simulink model "scenarioCloseLoop_supervisoryACC_start"  (R2019b)
settings: Solver=VariableStepAuto  StartTime=0.0  StopTime=30  FixedStep=0.01  RelTol=1e-3
PreLoadFcn:
  | Ts1 = -1;
  | Ts2 = -1;
InitFcn:
  | initACCParams_pid;
model workspace (MAT data in the model file):
  firstWarning = 1
  originalScenarioChecksum = '3C3E23DDE530CB8BEC76DD6DBB66960A'
undefined symbols (not defined in the file): APP_gain, BPP_gain, default_spacing, DiscIntNeverNeededParam, m, sigbuilder_block, steer_gain, time_gap
libraries: drivingscenarioandsensors x2, simulink x1, autolibshared x1, vehdynlibviscommon x1
settings Model: EnablePacing=on  Creator=sseshadr  LastModifiedBy=cdsouza
settings SolverCC: AutoInsertRateTranBlk=on
settings OptimizationCC: DefaultParameterBehavior=Inlined  EnhancedBackFolding=on  PassReuseOutputArgsThreshold=0  OptimizeBlockOrder=speed  DifferentSizesBufferReuse=on  OptimizationCustomize=off
settings DebuggingCC: ParameterTunabilityLossMsg=error
settings SFSimCC: MATLABDynamicMemAlloc=off
settings RTWCC: Description=Generic Real-Time Target  GenerateReport=on  LaunchReport=on
settings CodeAppCC: ForceParamTrailComments=on  OperatorAnnotations=on  StateflowObjectComments=on

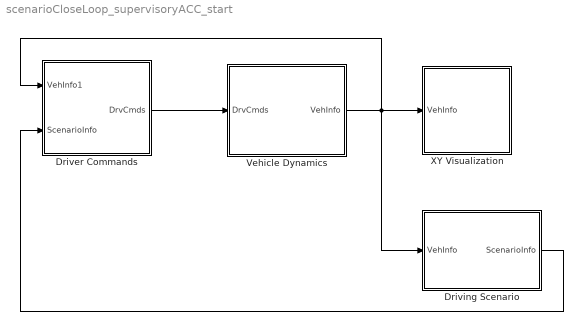
== system scenarioCloseLoop_supervisoryACC_start ==
  Driver Commands : Subsystem
  Driving Scenario : Subsystem
  Vehicle Dynamics : Subsystem
  XY Visualization : Subsystem
  wires:
  Driving Scenario/1(ScenarioInfo) -> Driver Commands/2(ScenarioInfo)
  Driver Commands/1(DrvCmds) -> Vehicle Dynamics/1(DrvCmds)
  Vehicle Dynamics/1(VehInfo) -> Driving Scenario/1(VehInfo), XY Visualization/1(VehInfo), Driver Commands/1(VehInfo1)

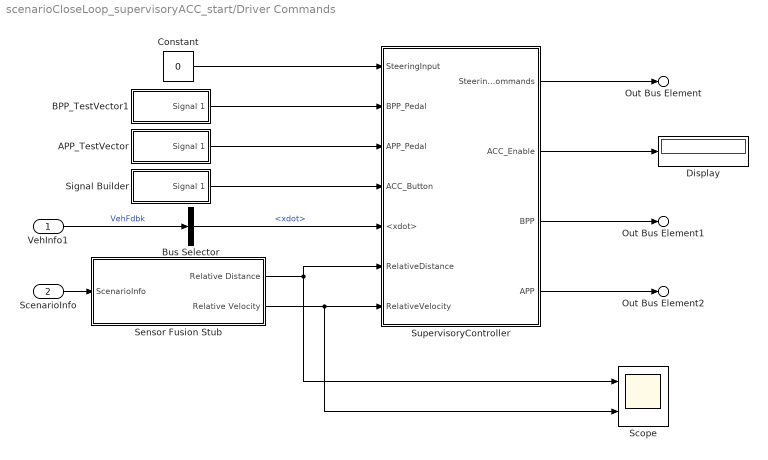
== system scenarioCloseLoop_supervisoryACC_start/Driver Commands ==
  VehInfo1 : Inport
  ScenarioInfo : Inport  Port=2
  APP_TestVector : Subsystem  Tag=STV Subsys  LoadFcn=sigbuilder_block('load');  StartFcn=sigbuilder_block('start');  StopFcn=sigbuilder_block('stop');  ClipboardFcn=sigbuilder_block('clipboard');  mask(Sigbuilder block){tuvar=[0:10]}
      mask help: Simulink:masks:SigbuilderBlock_MD
      mask init:
      | if ~strcmp(get_param(bdroot(gcbh),'SimulationStatus'),'stopped') tuvar = sigbuilder_block('maskInit'); end
      settings: CopyFcn=sigbuilder_block('copy');  DeleteFcn=sigbuilder_block('delete');  ModelCloseFcn=sigbuilder_block('modelClose');  PreSaveFcn=sigbuilder_block('preSave');  PauseFcn=sigbuilder_block('pause');  ContinueFcn=sigbuilder_block('continue');  NameChangeFcn=sigbuilder_block('namechange');  OpenFcn=sigbuilder_block('open',[609 515.25 550.5 237.75 ]);  CloseFcn=sigbuilder_block('close');
      mask Display: plot(0, 0, 100, 100,[2, 2, 32, 32, 2], [68, 8, 8, 68, 68],[32, 2], [38, 38], [32, 19, 2],[53, 60, 44], [32, 17, 17, 2],[16, 16, 31, 31]);txt = getActiveGroup(gcbh);text(2, 100, txt,'verticalAlignment', 'top');
  BPP_TestVector1 : Subsystem  Tag=STV Subsys  LoadFcn=sigbuilder_block('load');  StartFcn=sigbuilder_block('start');  StopFcn=sigbuilder_block('stop');  ClipboardFcn=sigbuilder_block('clipboard');  mask(Sigbuilder block){tuvar=[0:10]}
      mask help: Simulink:masks:SigbuilderBlock_MD
      mask init:
      | if ~strcmp(get_param(bdroot(gcbh),'SimulationStatus'),'stopped') tuvar = sigbuilder_block('maskInit'); end
      settings: CopyFcn=sigbuilder_block('copy');  DeleteFcn=sigbuilder_block('delete');  ModelCloseFcn=sigbuilder_block('modelClose');  PreSaveFcn=sigbuilder_block('preSave');  PauseFcn=sigbuilder_block('pause');  ContinueFcn=sigbuilder_block('continue');  NameChangeFcn=sigbuilder_block('namechange');  OpenFcn=sigbuilder_block('open',[325.5 304.5 550.5 278.25 ]);  CloseFcn=sigbuilder_block('close');
      mask Display: plot(0, 0, 100, 100,[2, 2, 32, 32, 2], [68, 8, 8, 68, 68],[32, 2], [38, 38], [32, 19, 2],[53, 60, 44], [32, 17, 17, 2],[16, 16, 31, 31]);txt = getActiveGroup(gcbh);text(2, 100, txt,'verticalAlignment', 'top');
  Bus Selector : BusSelector  OutputSignals=BdyFrm.Cg.Vel.xdot
  Constant : Constant  Value=0  SampleTime=0.01
  Display : Display
  Scope : Scope  NumInputPorts=2
  Sensor Fusion Stub : Subsystem
  Signal Builder : Subsystem  Tag=STV Subsys  LoadFcn=sigbuilder_block('load');  StartFcn=sigbuilder_block('start');  StopFcn=sigbuilder_block('stop');  ClipboardFcn=sigbuilder_block('clipboard');  mask(Sigbuilder block){tuvar=[0:10]}
      mask help: Simulink:masks:SigbuilderBlock_MD
      mask init:
      | if ~strcmp(get_param(bdroot(gcbh),'SimulationStatus'),'stopped') tuvar = sigbuilder_block('maskInit'); end
      settings: CopyFcn=sigbuilder_block('copy');  DeleteFcn=sigbuilder_block('delete');  ModelCloseFcn=sigbuilder_block('modelClose');  PreSaveFcn=sigbuilder_block('preSave');  PauseFcn=sigbuilder_block('pause');  ContinueFcn=sigbuilder_block('continue');  NameChangeFcn=sigbuilder_block('namechange');  OpenFcn=sigbuilder_block('open',[401.25 280.5 550.5 278.25 ]);  CloseFcn=sigbuilder_block('close');
      mask Display: plot(0, 0, 100, 100,[2, 2, 32, 32, 2], [68, 8, 8, 68, 68],[32, 2], [38, 38], [32, 19, 2],[53, 60, 44], [32, 17, 17, 2],[16, 16, 31, 31]);txt = getActiveGroup(gcbh);text(2, 100, txt,'verticalAlignment', 'top');
  SupervisoryController : Subsystem
  Out Bus Element : Outport  PortName=DrvCmds  Element=SteerCmd
  Out Bus Element1 : Outport  PortName=DrvCmds  Element=BPP Pedal
  Out Bus Element2 : Outport  PortName=DrvCmds  Element=APP Pedal
  wires:
  ScenarioInfo/1 -> Sensor Fusion Stub/1(ScenarioInfo)
  Sensor Fusion Stub/1(Relative Distance) -> SupervisoryController/6(RelativeDistance), Scope/1
  Sensor Fusion Stub/2(Relative Velocity) -> Scope/2, SupervisoryController/7(RelativeVelocity)
  SupervisoryController/1(SteeringCommands) -> Out Bus Element/1
  SupervisoryController/2(ACC_Enable) -> Display/1
  SupervisoryController/3(BPP) -> Out Bus Element1/1
  SupervisoryController/4(APP) -> Out Bus Element2/1
  Bus Selector/1 -> SupervisoryController/5(<xdot>)  "<xdot>"
  VehInfo1/1 -> Bus Selector/1  "VehFdbk"
  Signal Builder/1(Signal 1) -> SupervisoryController/4(ACC_Button)
  Constant/1 -> SupervisoryController/1("SteeringInput ")
  BPP_TestVector1/1(Signal 1) -> SupervisoryController/2(BPP_Pedal)
  APP_TestVector/1(Signal 1) -> SupervisoryController/3(APP_Pedal)

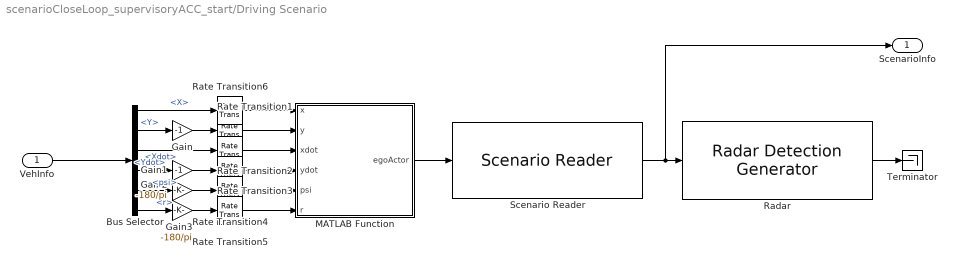
== system scenarioCloseLoop_supervisoryACC_start/Driving Scenario ==
  VehInfo : Inport
  Bus Selector : BusSelector  OutputSignals=InertFrm.Cg.Disp.X,InertFrm.Cg.Disp.Y,InertFrm.Cg.Vel.Xdot,InertFrm.Cg.Vel.Ydot,InertFrm.Cg.Ang.psi,BdyFrm.Cg.AngVel.r
  Gain : Gain  Gain=-1
  Gain1 : Gain  Gain=-1
  Gain2 : Gain  Gain=-180/pi
  Gain3 : Gain  Gain=-180/pi
  MATLAB Function : MATLAB Function  TreatAsAtomicUnit=on
  Radar : drivingscenarioandsensors/Radar Detection Generator  SensorIndex=1  UpdateInterval=0.1  SensorLocation=[3.5 0]  Height=0.2  Yaw=0  Pitch=0  Roll=0  BusNameSource=Auto  BusName=BusRadarDetectionGenerator  MaxNumDetectionsSource=Property  MaxNumDetections=50  DetectionCoordinates=Ego Cartesian  SimulateUsing=Interpreted execution  AzimuthResolution=4  ElevationResolution=10  RangeResolution=2.5  RangeRateResolution=0.5  AzimuthBiasFraction=0.1  ElevationBiasFraction=0.1  RangeBiasFraction=0.05  RangeRateBiasFraction=0.05  FieldOfView=[100 5]  MaxRange=50  RangeRateLimits=[-100 100]  DetectionProbability=0.9  FalseAlarmRate=1e-06  ReferenceRange=100  ReferenceRCS=0  HasElevation=off  HasRangeRate=on  HasNoise=on  HasFalseAlarms=on  HasOcclusion=on  InitialSeedSource=Repeatable  InitialSeed=0  UsedSeed=0  ActorProfilesSource=MATLAB expression  ActorProfilesParameters=driving.internal.ActorProfilesRadarParameters  ActorProfilesExpression=[struct('ActorID',1,'ClassID',1,'Length',4.7,'Width',1.8,'Height',1.4,'OriginOffset',[-1.35 0 0],'RCSPattern',[10 10;10 10],'RCSAzimuthAngles',[-180 180],'RCSElevationAngles',[-90 90]); struct('ActorID',2,'ClassID',1,'Length',4.7,'Width',1.8,'Height',1.4,'OriginOffset',[-1.35 0 0],'RCSPattern',[10 10;10 10],'RCSAzimuthAngles',[-180 180],'RCSElevationAngles',[-90 90]); struct('ActorID',3,'ClassID',1,'Length',4.7,'Width',1.8,'Height',1.4,'OriginOffset',[-1.35 0 0],'RCSPattern',[10 10;10 10],'RCSAzimuthAngles',[-180 180],'RCSElevationAngles',[-90 90]); struct('ActorID',4,'ClassID',1,'Length',4.7,'Width',1.8,'Height',1.4,'OriginOffset',[-1.35 0 0],'RCSPattern',[10 10;10 10],'RCSAzimuthAngles',[-180 180],'RCSElevationAngles',[-90 90])]
      settings: SourceProductName=Automated Driving Toolbox  SourceProductBaseCode=DR
  Rate Transition{1..6} (6 alike) : RateTransition  OutPortSampleTime=0.1
  Scenario Reader : drivingscenarioandsensors/Scenario Reader  ScenarioSource=From file  ScenarioFileName=Straight.mat  ScenarioVariableName=scenario  OutputCoordinateSystem=Vehicle coordinates  EgoVehicleSource=Input port  EgoVehicleActorID=1  SampleTime=0.1  LaneBoundaryOutput=None  LaneBoundaryDistance=0:0.5:9.5  LaneBoundaryLocation=Center of lane markings  BusNameSource=Auto  BusName=BusActors  BusName2Source=Auto  BusName2=BusLaneBoundaries  SimulateUsing=Interpreted execution
      settings: SourceProductName=Automated Driving Toolbox
  Terminator : Terminator
  ScenarioInfo : Outport
  wires:
  Bus Selector/3 -> Rate Transition2/1  "<Xdot>"
  Bus Selector/6 -> Gain3/1  "<r>"
  Bus Selector/1 -> Rate Transition6/1  "<X>"
  Bus Selector/2 -> Gain/1  "<Y>"
  Bus Selector/5 -> Gain2/1  "<psi>"
  VehInfo/1 -> Bus Selector/1
  Bus Selector/4 -> Gain1/1  "<Ydot>"
  Rate Transition6/1 -> MATLAB Function/1(x)
  Rate Transition1/1 -> MATLAB Function/2(y)
  Rate Transition2/1 -> MATLAB Function/3(xdot)
  Rate Transition3/1 -> MATLAB Function/4(ydot)
  Rate Transition4/1 -> MATLAB Function/5(psi)
  Rate Transition5/1 -> MATLAB Function/6(r)
  Radar/1 -> Terminator/1
  Scenario Reader/1 -> ScenarioInfo/1, Radar/1
  MATLAB Function/1(egoActor) -> Scenario Reader/1
  Gain/1 -> Rate Transition1/1
  Gain1/1 -> Rate Transition3/1
  Gain2/1 -> Rate Transition4/1
  Gain3/1 -> Rate Transition5/1

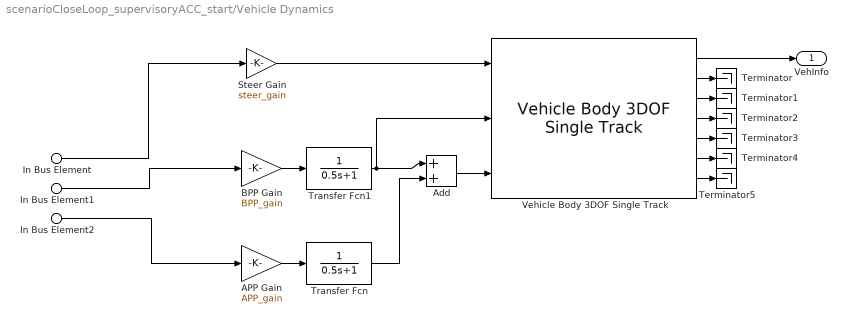
== system scenarioCloseLoop_supervisoryACC_start/Vehicle Dynamics ==
  In Bus Element : Inport  PortName=DrvCmds  Element=SteerCmd
  In Bus Element1 : Inport  PortName=DrvCmds  Element=BPP Pedal
  In Bus Element2 : Inport  PortName=DrvCmds  Element=APP Pedal
  APP Gain : Gain  Gain=APP_gain
  Add : Sum
  BPP Gain : Gain  Gain=BPP_gain
  Steer Gain : Gain  Gain=steer_gain
  Terminator{,1..5} (6 alike) : Terminator
  Transfer Fcn : TransferFcn  Denominator=[0.5 1]
  Transfer Fcn1 : TransferFcn  Denominator=[0.5 1]
  Vehicle Body 3DOF Single Track : autolibshared/Vehicle Body 3DOF Single Track  trackMode=Single (bicycle)  inputMode=External longitudinal forces  frontSteerMode=on  rearSteerMode=off  windMode=off  muMode=off  extFMode=off  extMMode=off  extXo=off  extpsio=off  extxdoto=off  extro=off  extYo=off  extTamb=off  extydoto=off  aMode=2  NF=2  NR=2  m=m  a=1.4  b=1.6  h=0.35  X_o=0  xdot_o=0  CalphaMode=off  sigmaMode=on  d=0  w=[1.4,1.4]  Cy_f=12e3  Cy_r=11e3  sigma_f=.1  sigma_r=.1  alpha_f_brk=[-.1 .1]  Cy_f_data=[-9e3 9e3]  alpha_r_brk=[-.1 .1]  Cy_r_data=[-9e3 9e3]  Y_o=0  ydot_o=0  Izz=4000  psi_o=0  r_o=0  Af=2  Cd=.3  Cl=.1  Cpm=.1  beta_w=[0:0.01:0.3]  Cs=[0:0.03:0.9]  Cym=[0:0.01:0.3]  Pabs=101325  Tair=273  g=9.81  mu=1  xdot_tol=.01  Fznom=5000  Fxtire_sat=7e4  Fytire_sat=7e4  longOff=0  latOff=0  vertOff=0  wrapAng=off
      settings: SourceProductName=Powertrain Blockset  SourceProductBaseCode=PW
  VehInfo : Outport
  wires:
  Vehicle Body 3DOF Single Track/7 -> Terminator5/1
  Transfer Fcn/1 -> Add/2
  Vehicle Body 3DOF Single Track/6 -> Terminator4/1
  BPP Gain/1 -> Transfer Fcn1/1
  In Bus Element1/1 -> BPP Gain/1
  Steer Gain/1 -> Vehicle Body 3DOF Single Track/1
  Vehicle Body 3DOF Single Track/4 -> Terminator2/1
  Vehicle Body 3DOF Single Track/2 -> Terminator/1
  Vehicle Body 3DOF Single Track/5 -> Terminator3/1
  Transfer Fcn1/1 -> Vehicle Body 3DOF Single Track/2, Add/1
  APP Gain/1 -> Transfer Fcn/1
  Vehicle Body 3DOF Single Track/3 -> Terminator1/1
  Add/1 -> Vehicle Body 3DOF Single Track/3
  Vehicle Body 3DOF Single Track/1 -> VehInfo/1
  In Bus Element/1 -> Steer Gain/1
  In Bus Element2/1 -> APP Gain/1

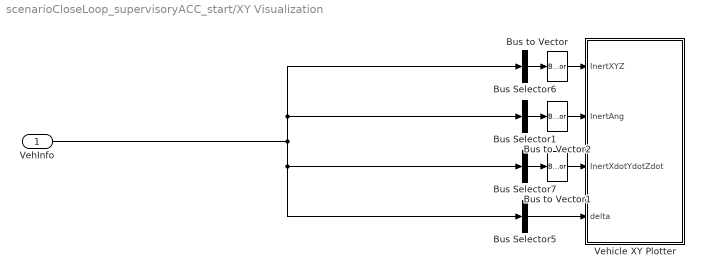
== system scenarioCloseLoop_supervisoryACC_start/XY Visualization ==
  VehInfo : Inport
  Bus Selector1 : BusSelector  OutputSignals=InertFrm.Cg.Ang.phi,InertFrm.Cg.Ang.theta,InertFrm.Cg.Ang.psi  OutputAsBus=on
  Bus Selector5 : BusSelector  OutputSignals=BdyFrm.FrntAxl.Steer.WhlAngFL,BdyFrm.FrntAxl.Steer.WhlAngFR,BdyFrm.RearAxl.Steer.WhlAngRL,BdyFrm.RearAxl.Steer.WhlAngRR  OutputAsBus=on
  Bus Selector6 : BusSelector  OutputSignals=InertFrm.Geom.Disp.X,InertFrm.Geom.Disp.Y,InertFrm.Geom.Disp.Z  OutputAsBus=on
  Bus Selector7 : BusSelector  OutputSignals=InertFrm.Geom.Vel.Xdot,InertFrm.Geom.Vel.Ydot,InertFrm.Geom.Vel.Zdot  OutputAsBus=on
  Bus to Vector : BusToVector
  Bus to Vector1 : BusToVector
  Bus to Vector2 : BusToVector
  Vehicle XY Plotter : Subsystem  mask(Vehicle XY Plotter){a=2, b=2, w=2, figBorder=10, bufferSize=1024, extRef=off, pltDT=.1}
      mask prompts: a "Distance to front axle from CG, a [m]:"; b "Distance to rear axle from CG, b [m]:"; w "Track width, w [m]:"; figBorder "Distance to figure borders, figBorder [m]:"; bufferSize "Path buffer sampe size, bufferSize []:"; extRef "Plot path reference, extRef"; pltDT "Plot update rate, pltDT [s]:"
      mask help:
      | This block will display a MATLAB figure which indicates the vehicle path, current position and heading velocity.
      | An optional path reference is also provided.
      mask init:
      | if autoblkschecksimstopped(gcb)
      |     PortName = 'RefXYZ';
      |     InportOption  = {'built-in/Ground', [PortName, ' Ground'];...
      |         'built-in/Inport',PortName };
      |     if ~strcmp(get_param(gcb,'extRef'),'on')
      |         NewBlkHdl = autoblksreplaceblock(gcb, InportOption, 1);
      |         set_param(NewBlkHdl, 'ShowName', 'off');
      |     else
      |         autoblksreplaceblock(gcb, InportOption, 2);
      |     end
      | end
      mask TypeOptions a: Vehicle XY Plotter/a
      mask TypeOptions b: Vehicle XY Plotter/b
      mask TypeOptions w: Vehicle XY Plotter/w
      mask TypeOptions figBorder: Vehicle XY Plotter/figBorder
      mask TypeOptions bufferSize: Vehicle XY Plotter/bufferSize
  wires:
  Bus Selector5/1 -> Vehicle XY Plotter/4(delta)
  Bus Selector7/1 -> Bus to Vector1/1
  Bus Selector6/1 -> Bus to Vector/1
  Bus to Vector2/1 -> Vehicle XY Plotter/2(InertAng)
  Bus Selector1/1 -> Bus to Vector2/1
  Bus to Vector/1 -> Vehicle XY Plotter/1(InertXYZ)
  Bus to Vector1/1 -> Vehicle XY Plotter/3(InertXdotYdotZdot)
  VehInfo/1 -> Bus Selector5/1, Bus Selector7/1, Bus Selector6/1, Bus Selector1/1

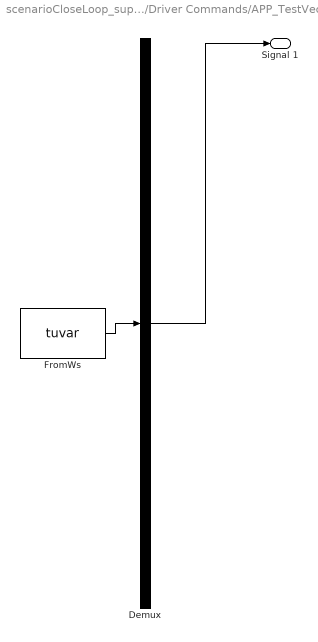
== system scenarioCloseLoop_supervisoryACC_start/Driver Commands/APP_TestVector ==
  Demux : Demux  Tag=STV Demux  Outputs=1
  FromWs : FromWorkspace  Tag=STV FromWs  VariableName=tuvar  SampleTime=0
      SigBuilderData=|
      | common.afterFinalStr = 'Extrapolate'
      | common.sampleTime = 0
      | dataSet.timeRange = [0 10]
      | dataSet.name = 'Group 1'
      | sbobj.Groups.Name = 'Group 1'
      | sbobj.Groups.Signals.Name = 'Signal 1'
      | sbobj.Groups.Signals.XData = [0 1 2 2.2 4 6 10]
      | sbobj.Groups.Signals.YData = [0.8 0.19 0.6 0 0 0 0]
  Signal 1 : Outport  Tag=STV Outport
  wires:
  FromWs/1 -> Demux/1
  Demux/1 -> Signal 1/1

== system scenarioCloseLoop_supervisoryACC_start/Driver Commands/BPP_TestVector1 ==
  Demux : Demux  Tag=STV Demux  Outputs=1
  FromWs : FromWorkspace  Tag=STV FromWs  VariableName=tuvar  SampleTime=0
      SigBuilderData=|
      | common.afterFinalStr = 'Extrapolate'
      | common.sampleTime = 0
      | dataSet.timeRange = [0 10]
      | dataSet.name = 'Group 1'
      | sbobj.Groups.Name = 'Group 1'
      | sbobj.Groups.Signals.Name = 'Signal 1'
      | sbobj.Groups.Signals.XData = [0 1 2 2.2 4 6 10]
      | sbobj.Groups.Signals.YData = [0 0.4 0 0 0 0 0]
  Signal 1 : Outport  Tag=STV Outport
  wires:
  Demux/1 -> Signal 1/1
  FromWs/1 -> Demux/1

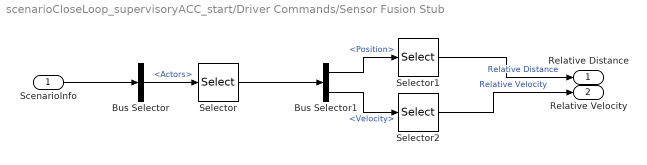
== system scenarioCloseLoop_supervisoryACC_start/Driver Commands/Sensor Fusion Stub ==
  ScenarioInfo : Inport
  Bus Selector : BusSelector  OutputSignals=Actors
  Bus Selector1 : BusSelector  OutputSignals=Position,Velocity
  Selector : Selector  InputPortWidth=3  IndexOptions=Index vector (dialog)  Indices=3  OutputSizes=1
  Selector1 : Selector  InputPortWidth=3  IndexOptions=Index vector (dialog)  Indices=1  OutputSizes=1
  Selector2 : Selector  InputPortWidth=3  IndexOptions=Index vector (dialog)  Indices=1  OutputSizes=1
  Relative Distance : Outport
  Relative Velocity : Outport  Port=2
  wires:
  Selector/1 -> Bus Selector1/1
  Selector2/1 -> Relative Velocity/1  "Relative Velocity"
  ScenarioInfo/1 -> Bus Selector/1
  Bus Selector/1 -> Selector/1  "<Actors>"
  Selector1/1 -> Relative Distance/1  "Relative Distance"
  Bus Selector1/1 -> Selector1/1  "<Position>"
  Bus Selector1/2 -> Selector2/1  "<Velocity>"

== system scenarioCloseLoop_supervisoryACC_start/Driver Commands/Signal Builder ==
  Demux : Demux  Tag=STV Demux  Outputs=1
  FromWs : FromWorkspace  Tag=STV FromWs  VariableName=tuvar  SampleTime=0
      SigBuilderData=|
      | common.afterFinalStr = 'Extrapolate'
      | common.sampleTime = 0
      | dataSet.timeRange = [0 10]
      | dataSet.name = 'Group 1'
      | sbobj.Groups.Name = 'Group 1'
      | sbobj.Groups.Signals.Name = 'Signal 1'
      | sbobj.Groups.Signals.XData = [0 2.15 2.15 2.2 2.2 4 6 6 10]
      | sbobj.Groups.Signals.YData = [-1 -1 180 180 -1 -1 1 0 0]
  Signal 1 : Outport  Tag=STV Outport
  wires:
  Demux/1 -> Signal 1/1
  FromWs/1 -> Demux/1

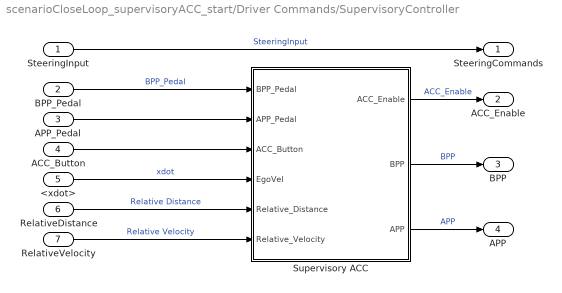
== system scenarioCloseLoop_supervisoryACC_start/Driver Commands/SupervisoryController ==
  "SteeringInput " : Inport  OutDataTypeStr=double  PortDimensions=1  SampleTime=Ts1
  BPP_Pedal : Inport  Port=2  OutDataTypeStr=double  PortDimensions=1  SampleTime=Ts1
  APP_Pedal : Inport  Port=3  OutDataTypeStr=double  PortDimensions=1  SampleTime=Ts1
  ACC_Button : Inport  Port=4  OutDataTypeStr=double  PortDimensions=1  SampleTime=Ts1
  <xdot> : Inport  Port=5  OutDataTypeStr=double  PortDimensions=1  SampleTime=Ts1
  RelativeDistance : Inport  Port=6  OutDataTypeStr=double  PortDimensions=[1 1]  SampleTime=Ts2
  RelativeVelocity : Inport  Port=7  OutDataTypeStr=double  PortDimensions=[1 1]  SampleTime=Ts2
  Supervisory ACC : Stateflow chart  BlockKeywords=__PRM__SERIALIZED__DATA__:Stateflow Chart,Stateflow Diagram
  SteeringCommands : Outport  OutDataTypeStr=double  PortDimensions=1
  ACC_Enable : Outport  Port=2  OutDataTypeStr=double  PortDimensions=1
  BPP : Outport  Port=3  OutDataTypeStr=double  PortDimensions=1
  APP : Outport  Port=4  OutDataTypeStr=double  PortDimensions=1
  wires:
  APP_Pedal/1 -> Supervisory ACC/2(APP_Pedal)
  Supervisory ACC/1(ACC_Enable) -> ACC_Enable/1  "ACC_Enable"
  RelativeVelocity/1 -> Supervisory ACC/6(Relative_Velocity)  "Relative Velocity"
  Supervisory ACC/3(APP) -> APP/1  "APP"
  ACC_Button/1 -> Supervisory ACC/3(ACC_Button)
  "SteeringInput "/1 -> SteeringCommands/1  "SteeringInput"
  <xdot>/1 -> Supervisory ACC/4(EgoVel)  "xdot"
  Supervisory ACC/2(BPP) -> BPP/1  "BPP"
  BPP_Pedal/1 -> Supervisory ACC/1(BPP_Pedal)  "BPP_Pedal"
  RelativeDistance/1 -> Supervisory ACC/5(Relative_Distance)  "Relative Distance"

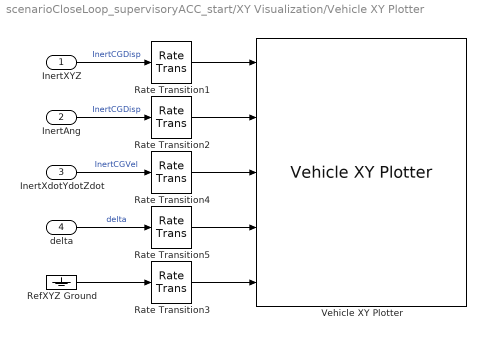
== system scenarioCloseLoop_supervisoryACC_start/XY Visualization/Vehicle XY Plotter ==
  InertXYZ : Inport
  InertAng : Inport  Port=2
  InertXdotYdotZdot : Inport  Port=3
  delta : Inport  Port=4
  Rate Transition{1..5} (5 alike) : RateTransition  Deterministic=off  OutPortSampleTime=pltDT
  RefXYZ Ground : Ground
  Vehicle XY Plotter : vehdynlibviscommon/Vehicle XY Plotter  bufferSize=bufferSize  w=w  a=a  b=b  figBorder=figBorder
      settings: SourceProductName=Vehicle Dynamics Blockset  SourceProductBaseCode=VE
  wires:
  Rate Transition5/1 -> Vehicle XY Plotter/4
  Rate Transition4/1 -> Vehicle XY Plotter/3
  Rate Transition2/1 -> Vehicle XY Plotter/2
  Rate Transition1/1 -> Vehicle XY Plotter/1
  Rate Transition3/1 -> Vehicle XY Plotter/5
  delta/1 -> Rate Transition5/1  "delta"
  InertXYZ/1 -> Rate Transition1/1  "InertCGDisp"
  InertXdotYdotZdot/1 -> Rate Transition4/1  "InertCGVel"
  InertAng/1 -> Rate Transition2/1  "InertCGDisp"
  RefXYZ Ground/1 -> Rate Transition3/1

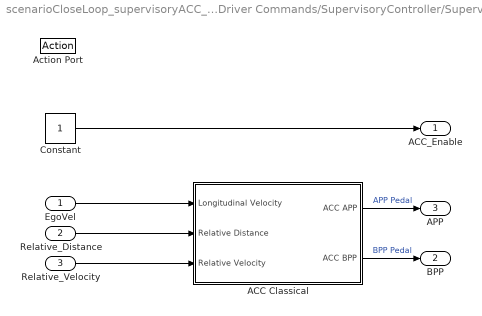
== system scenarioCloseLoop_supervisoryACC_start/Driver Commands/SupervisoryController/Supervisory ACC/ACC ==
  EgoVel : Inport
  Relative_Distance : Inport  Port=2
  Relative_Velocity : Inport  Port=3
  Action Port : ActionPort
      settings: CopyFcn=Stateflow.SLINSF.SimulinkMan.removeBlockPreDeleteFcn  PreDeleteFcn=Stateflow.SLINSF.SimulinkMan.unsafePredeleteFcn
  ACC Classical : Subsystem  VariantControl=controller_type == 1
      settings: RTWFileNameOpts=Use function name
  Constant : Constant  SampleTime=-1
  ACC_Enable : Outport
  BPP : Outport  Port=2
  APP : Outport  Port=3
  wires:
  Constant/1 -> ACC_Enable/1
  ACC Classical/2(ACC BPP) -> BPP/1  "BPP Pedal"
  ACC Classical/1(ACC APP) -> APP/1  "APP Pedal"
  Relative_Velocity/1 -> ACC Classical/3(Relative Velocity)
  Relative_Distance/1 -> ACC Classical/2(Relative Distance)
  EgoVel/1 -> ACC Classical/1(Longitudinal Velocity)

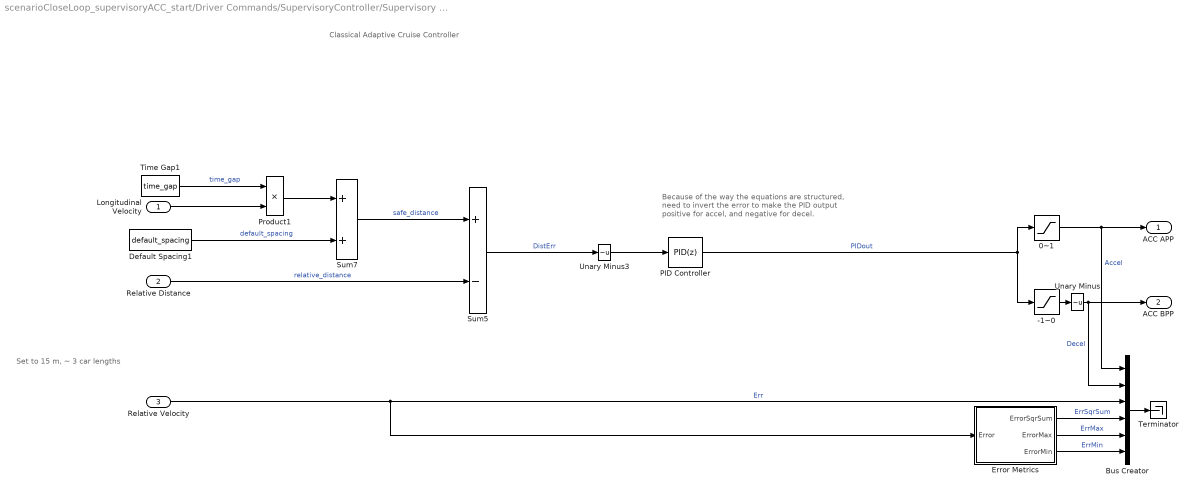
== system scenarioCloseLoop_supervisoryACC_start/Driver Commands/SupervisoryController/Supervisory ACC/ACC/ACC Classical ==
  note: Classical Adaptive Cruise Controller
  note: Set to 15 m, ~ 3 car lengths
  note: Because of the way the equations are structured,
      | need to invert the error to make the PID output
      | positive for accel, and negative for decel.
  Longitudinal Velocity : Inport
  Relative Distance : Inport  Port=2
  Relative Velocity : Inport  Port=3
  -1~0 : Saturate  UpperLimit=0  LowerLimit=-1  ZeroCross=off
  0~1 : Saturate  UpperLimit=1  LowerLimit=0  ZeroCross=off
  Bus Creator : BusCreator  Inputs=6
  Default Spacing1 : Constant  Value=default_spacing  SampleTime=-1
  Error Metrics : Subsystem
  PID Controller : simulink/Continuous/PID Controller  Controller=PID  Form=Parallel  TimeDomain=Discrete-time  SampleTime=-1  IntegratorMethod=Forward Euler  FilterMethod=Forward Euler  ControllerParametersSource=internal  P=0.05  I=0.001  D=0.05  UseFilter=on  N=10  TunerSelectOption=Transfer Function Based (PID Tuner App)  InitialConditionSource=internal  InitialConditionForIntegrator=0  InitialConditionForFilter=0  DifferentiatorICPrevScaledInput=0  ExternalReset=none  TrackingMode=off  Kt=1  LimitOutput=on  UpperSaturationLimit=1  LowerSaturationLimit=-1  LinearizeAsGain=on  AntiWindupMode=clamping  Kb=1  POutMin=[]  POutMax=[]  IOutMin=[]  IOutMax=[]  DOutMin=[]  DOutMax=[]  NOutMin=[]  NOutMax=[]  SumOutMin=[]  SumOutMax=[]  SaturationOutMin=[]  SaturationOutMax=[]  PParamMin=[]  PParamMax=[]  IParamMin=[]  IParamMax=[]  DParamMin=[]  DParamMax=[]  NParamMin=[]  NParamMax=[]  KbParamMin=[]  KbParamMax=[]  KtParamMin=[]  KtParamMax=[]  KbOutMin=[]  KbOutMax=[]  KtOutMin=[]  KtOutMax=[]  IntegratorOutMin=[]  IntegratorOutMax=[]  FilterOutMin=[]  FilterOutMax=[]  SumI1OutMin=[]  SumI1OutMax=[]  SumI2OutMin=[]  SumI2OutMax=[]  SumI3OutMin=[]  SumI3OutMax=[]  SumI4OutMin=[]  SumI4OutMax=[]  SumDOutMin=[]  SumDOutMax=[]  DifferentiatorOutMin=[]  DifferentiatorOutMax=[]  FilterDiffOutCoefMin=[]  FilterDiffOutCoefMax=[]  ReciprocalOutMin=[]  ReciprocalOutMax=[]  SumDenOutMin=[]  SumDenOutMax=[]  SumNumOutMin=[]  SumNumOutMax=[]  DivideOutMin=[]  DivideOutMax=[]  IntegratorContinuousStateAttributes=''  IntegratorStateMustResolveToSignalObject=off  IntegratorRTWStateStorageClass=Auto  FilterContinuousStateAttributes=''  FilterStateMustResolveToSignalObject=off  FilterRTWStateStorageClass=Auto  ParallelPVariant=InternalParameters  IdealPVariant=Disabled  IVariant=InternalParameters  DVariant=InternalParameters  IntegratorVariant=Discrete  SatVariant=Enabled  AWVariant=DiscClampingParallel  PCopyVariant=Disabled  TRVariant=Disabled  FdbkBlocksVariant=Forward  IdealPFdbkVariant=Disabled  SatFdbkVariant=Disabled  DerivativeFilterVariant=ForwardEulerFilter  NVariant=InternalParameters  NCopyVariant=Disabled  FilterICVariant=InternalICsFilter  IntegratorICVariant=InternalICs  ExternalResetVariant=Disabled  TRSumVariant=Passthrough  SumFdbkVariant=Disabled  SumVariant=Sum_PID
  Product1 : Product
  Sum5 : Sum  Inputs=+-
  Sum7 : Sum
  Terminator : Terminator
  Time Gap1 : Constant  Value=time_gap  SampleTime=-1
  Unary Minus : UnaryMinus
  Unary Minus3 : UnaryMinus
  ACC APP : Outport  Unit=one  InitialOutput=0  VectorParamsAs1DForOutWhenUnconnected=off
  ACC BPP : Outport  Port=2  Unit=one  InitialOutput=0  VectorParamsAs1DForOutWhenUnconnected=off
  wires:
  Error Metrics/2(ErrorMax) -> Bus Creator/5  "ErrMax"
  Default Spacing1/1 -> Sum7/2  "default_spacing"
  Sum7/1 -> Sum5/1  "safe_distance"
  Sum5/1 -> Unary Minus3/1  "DistErr"
  Unary Minus/1 -> Bus Creator/2, ACC BPP/1  "Decel"
  Product1/1 -> Sum7/1
  Relative Distance/1 -> Sum5/2  "relative_distance"
  Longitudinal Velocity/1 -> Product1/2
  Bus Creator/1 -> Terminator/1
  0~1/1 -> ACC APP/1, Bus Creator/1  "Accel"
  Time Gap1/1 -> Product1/1  "time_gap"
  Error Metrics/1(ErrorSqrSum) -> Bus Creator/4  "ErrSqrSum"
  -1~0/1 -> Unary Minus/1
  PID Controller/1 -> -1~0/1, 0~1/1  "PIDout"
  Unary Minus3/1 -> PID Controller/1
  Relative Velocity/1 -> Bus Creator/3, Error Metrics/1(Error)  "Err"
  Error Metrics/3(ErrorMin) -> Bus Creator/6  "ErrMin"

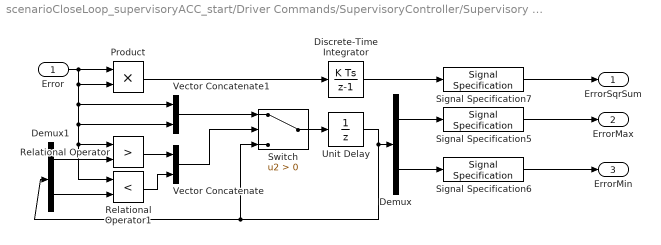
== system scenarioCloseLoop_supervisoryACC_start/Driver Commands/SupervisoryController/Supervisory ACC/ACC/ACC Classical/Error Metrics ==
  Error : Inport
  Demux : Demux  Outputs=2
  Demux1 : Demux  Outputs=2
  Discrete-Time Integrator : DiscreteIntegrator  SampleTime=-1  ICPrevOutput=DiscIntNeverNeededParam  ICPrevScaledInput=DiscIntNeverNeededParam
  Product : Product
  Relational Operator : RelationalOperator  Operator=>  OutDataTypeStr=boolean  ZeroCross=off  RndMeth=Simplest
  Relational Operator1 : RelationalOperator  Operator=<  OutDataTypeStr=boolean  ZeroCross=off  RndMeth=Simplest
  Signal Specification5 : SignalSpecification  Unit=m/s
  Signal Specification6 : SignalSpecification  Unit=m/s
  Signal Specification7 : SignalSpecification  Unit=m^2/s^2
  Switch : Switch  Criteria=u2 > Threshold
  Unit Delay : UnitDelay  InitialCondition=[0,0]  SampleTime=-1  HasFrameUpgradeWarning=on
  Vector Concatenate : Concatenate
  Vector Concatenate1 : Concatenate
  ErrorSqrSum : Outport  VectorParamsAs1DForOutWhenUnconnected=off
  ErrorMax : Outport  Port=2  VectorParamsAs1DForOutWhenUnconnected=off
  ErrorMin : Outport  Port=3  VectorParamsAs1DForOutWhenUnconnected=off
  wires:
  Discrete-Time Integrator/1 -> Signal Specification7/1
  Product/1 -> Discrete-Time Integrator/1
  Error/1 -> Product/2, Vector Concatenate1/2, Relational Operator1/1, Relational Operator/1, Vector Concatenate1/1, Product/1
  Switch/1 -> Unit Delay/1
  Unit Delay/1 -> Switch/3, Demux1/1, Demux/1
  Relational Operator1/1 -> Vector Concatenate/2
  Relational Operator/1 -> Vector Concatenate/1
  Vector Concatenate1/1 -> Switch/1
  Demux/1 -> Signal Specification5/1
  Demux/2 -> Signal Specification6/1
  Demux1/2 -> Relational Operator1/2
  Demux1/1 -> Relational Operator/2
  Vector Concatenate/1 -> Switch/2
  Signal Specification7/1 -> ErrorSqrSum/1
  Signal Specification6/1 -> ErrorMin/1
  Signal Specification5/1 -> ErrorMax/1

== matlab function scenarioCloseLoop_supervisoryACC_start/Driving Scenario/MATLAB Function ==
  data: x input; egoActor output Bus: BusActors1Actors; y input; xdot input; ydot input; psi input; r input
function egoActor = packActor(x,y,xdot,ydot,psi,r)

egoActor = struct(...
    'ActorID',1,...
    'Position', [x y 0], ...
    'Velocity', [xdot ydot 0], ...
    'Roll', 0, ...
    'Pitch', 0, ...
    'Yaw', psi, ...
    'AngularVelocity', [0 0 r]);

== stateflow chart scenarioCloseLoop_supervisoryACC_start/Driver Commands/SupervisoryController/Supervisory ACC ==
  state WaitOff
  state Normal
    during:
    APP = APP_Pedal;
    BPP = BPP_Pedal;
    ACC_Enable = 0;
  state ACC
  state WaitOn
  WaitOff -> Normal : [ACC_Button == -1]
  ACC -> WaitOff [order 2] : [ACC_Button == 180]
  (default) -> Normal
  ACC -> Normal [order 1] : [APP_Pedal || BPP_Pedal > 0]
  WaitOn -> ACC : [ACC_Button == -1]
  Normal -> WaitOn : [ACC_Button == 180]
  data: sf_internal_action_state_placeholder_data local double size=1 =0; ACC_Enable output; BPP output; APP output; BPP_Pedal input; APP_Pedal input; ACC_Button input; EgoVel input; Relative_Distance input; Relative_Velocity input
